simulink model "Assignment1"  (R2020a)
settings: Solver=FixedStepAuto  StartTime=0.0  StopTime=5  FixedStep=1e-3  RelTol=1e-3  EnableMultiTasking=on
model workspace (MAT data in the model file):
  ATR_CMP_REF_PWM_PERCENTAGE = 50
  PACING_REF_PWM_DUTY_PERCENTAGE = 50
  VENT_CMP_REF_PWM_PERCENTAGE = 50
undefined symbols (not defined in the file): A0, A1, D0, D1, D10, D11, D12, D13, D2, D3, D4, D5, D6, D7, D8, D9, magnitude, PTA0, PTA1, PTA2, PTB2, PTB23, PTB3, PTB9, PTC16, PTC17, PTC2, PTC3, PTC4, PTD0, PTD1, PTD2, PTD3
libraries: frdmk64flib x22, etargetslib x18, dspstat3 x1
settings Model: ExtModeTrigDuration=5  OrderedModelArguments=off  Creator=John  LastModifiedBy=changhaibian
settings OptimizationCC: EnhancedBackFolding=on  PassReuseOutputArgsAs=Individual arguments  ZeroExternalMemoryAtStartup=off  ZeroInternalMemoryAtStartup=off  MaxStackSize=64  OptimizeBlockOrder=speed  DifferentSizesBufferReuse=on  OptimizationCustomize=off  EfficientTunableParamExpr=on
settings DebuggingCC: ParameterTunabilityLossMsg=error
settings HardwareCC: ProdBitPerPointer=32  ProdBitPerSizeT=32  ProdBitPerPtrDiffT=32  ProdLargestAtomicInteger=Long  ProdLargestAtomicFloat=Double  ProdWordSize=32  ProdHWDeviceType=ARM Compatible->ARM Cortex
settings SFSimCC: MATLABDynamicMemAlloc=off
settings RTWCC: SystemTargetFile=ert.tlc  HardwareBoard=NXP FRDM-K64F  TemplateMakefile=ert_default_tmf  Toolchain=GNU Tools for ARM Embedded Processors
settings CodeAppCC: ForceParamTrailComments=on  IgnoreCustomStorageClasses=off  OperatorAnnotations=on  SimulinkDataObjDesc=on  SFDataObjDesc=on  InsertBlockDesc=on

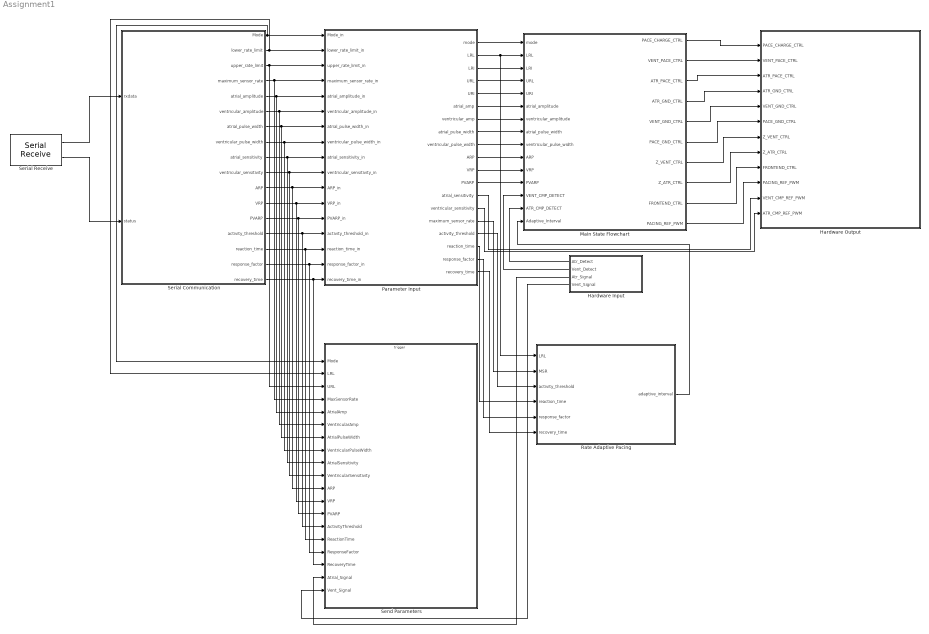
== system Assignment1 ==
  Hardware Input : Subsystem
      settings: PortSchema="{\"entries\":[{\"content\":{\"sides\":[{\"content\":{\"connectorIds\":[\"Out1\",\"Out2\",\"Out3\",\"Out4\"]},\"type\":\"ConnectorPlacement.EquallySpacedRectSide\",\"uuid\":\"5cee9ea6-bf5d-4625-bfce-39977475e911\"},{\"content\":{\"connectorIds\":[],\"side\":\"RIGHT\"},\"type\":\"ConnectorPlacement.EquallySpacedRectSide\",\"uuid\":\"d8f9e342-4161-4713-ba8e-977d0ac6df9e\"},{\"content\":{\"connectorIds\":[],\"side\":\"TOP\"},\"type\":\"ConnectorPlacement.EquallySpacedRectSide\",\"uuid\":\"5d530249-14f9-42e8-9a17-4b94b2159c30\"}]},\"type\":\"ConnectorPlacement.EquallySpacedConnector\",\"uuid\":\"d67ebefe-f0b3-4c88-9ae8-796034241cb9\"}],\"packageUris\":[\"http://schema.mathworks.com/mf0/Connector/19700101\"],\"version\":\"1.0\"}"
  Hardware Output : Subsystem
  Main State Flowchart : Stateflow chart  TreatAsAtomicUnit=on
  Parameter Input : Subsystem
  Rate Adaptive Pacing : Subsystem
  Send Parameters : Subsystem  TreatAsAtomicUnit=on
  Serial Communication : Stateflow chart  TreatAsAtomicUnit=on
  Serial Receive : frdmk64flib/Serial Receive  SCIModule=0  Baudrate=uint32(9600)  Parity=None  StopBits=1  HardwareFlowControl=None  ByteOrder=LittleEndian  DataType=uint8  DataLength=11  BlockingMode=off  OutputStatus=on  SampleTime=-1
  wires:
  Parameter Input/1(mode) -> Main State Flowchart/1(mode)
  Main State Flowchart/10(PACING_REF_PWM) -> Hardware Output/10(PACING_REF_PWM)
  Parameter Input/8(atrial_pulse_width) -> Main State Flowchart/8(atrial_pulse_width)
  Parameter Input/9(ventricular_pulse_width) -> Main State Flowchart/9(ventricular_pulse_width)
  Main State Flowchart/7(Z_VENT_CTRL) -> Hardware Output/7(Z_VENT_CTRL)
  Main State Flowchart/4(ATR_GND_CTRL) -> Hardware Output/4(ATR_GND_CTRL)
  Main State Flowchart/3(ATR_PACE_CTRL) -> Hardware Output/3(ATR_PACE_CTRL)
  Main State Flowchart/5(VENT_GND_CTRL) -> Hardware Output/5(VENT_GND_CTRL)
  Main State Flowchart/2(VENT_PACE_CTRL) -> Hardware Output/2(VENT_PACE_CTRL)
  Main State Flowchart/1(PACE_CHARGE_CTRL) -> Hardware Output/1(PACE_CHARGE_CTRL)
  Main State Flowchart/9(FRONTEND_CTRL) -> Hardware Output/9(FRONTEND_CTRL)
  Parameter Input/2(LRL) -> Rate Adaptive Pacing/1(LRL), Main State Flowchart/2(LRL)
  Parameter Input/10(ARP) -> Main State Flowchart/10(ARP)
  Parameter Input/11(VRP) -> Main State Flowchart/11(VRP)
  Parameter Input/6(atrial_amp) -> Main State Flowchart/6(atrial_amplitude)
  Parameter Input/3(LRI) -> Main State Flowchart/3(LRI)
  Parameter Input/4(URL) -> Main State Flowchart/4(URL)
  Parameter Input/5(URI) -> Main State Flowchart/5(URI)
  Serial Receive/1 -> Serial Communication/1(rxdata)
  Serial Receive/2 -> Serial Communication/2(status)
  Serial Communication/1(Mode) -> Send Parameters/1(Mode), Parameter Input/1(Mode_in)
  Serial Communication/2(lower_rate_limit) -> Send Parameters/2(LRL), Parameter Input/2(lower_rate_limit_in)
  Serial Communication/3(upper_rate_limit) -> Parameter Input/3(upper_rate_limit_in), Send Parameters/3(URL)
  Serial Communication/4(maximum_sensor_rate) -> Send Parameters/4(MaxSensorRate), Parameter Input/4(maximum_sensor_rate_in)
  Serial Communication/5(atrial_amplitude) -> Send Parameters/5(AtrialAmp), Parameter Input/5(atrial_amplitude_in)
  Serial Communication/6(ventricular_amplitude) -> Send Parameters/6(VentricularAmp), Parameter Input/6(ventricular_amplitude_in)
  Serial Communication/7(atrial_pulse_width) -> Send Parameters/7(AtrialPulseWidth), Parameter Input/7(atrial_pulse_width_in)
  Serial Communication/8(ventricular_pulse_width) -> Send Parameters/8(VentricularPulseWidth), Parameter Input/8(ventricular_pulse_width_in)
  Serial Communication/9(atrial_sensitivity) -> Send Parameters/9(AtrialSensitivity), Parameter Input/9(atrial_sensitivity_in)
  Serial Communication/10(ventricular_sensitivity) -> Send Parameters/10(VentricularSensitivity), Parameter Input/10(ventricular_sensitivity_in)
  Serial Communication/11(ARP) -> Send Parameters/11(ARP), Parameter Input/11(ARP_in)
  Serial Communication/12(VRP) -> Send Parameters/12(VRP), Parameter Input/12(VRP_in)
  Serial Communication/13(PVARP) -> Send Parameters/13(PVARP), Parameter Input/13(PVARP_in)
  Serial Communication/14(activity_threshold) -> Send Parameters/14(ActivityThreshold), Parameter Input/14(activity_threshold_in)
  Serial Communication/15(reaction_time) -> Send Parameters/15(ReactionTime), Parameter Input/15(reaction_time_in)
  Serial Communication/16(response_factor) -> Send Parameters/16(ResponseFactor), Parameter Input/16(response_factor_in)
  Serial Communication/17(recovery_time) -> Send Parameters/17(RecoveryTime), Parameter Input/17(recovery_time_in)
  Parameter Input/7(ventricular_amp) -> Main State Flowchart/7(ventricular_amplitude)
  Parameter Input/12(PVARP) -> Main State Flowchart/12(PVARP)
  Hardware Input/1(Atr_Detect) -> Main State Flowchart/14(ATR_CMP_DETECT)
  Hardware Input/2(Vent_Detect) -> Main State Flowchart/13(VENT_CMP_DETECT)
  Rate Adaptive Pacing/1(adaptive_interval) -> Main State Flowchart/15(Adaptive_Interval)
  Parameter Input/13(atrial_sensitivity) -> Hardware Output/11(VENT_CMP_REF_PWM)
  Parameter Input/14(ventricular_sensitivity) -> Hardware Output/12(ATR_CMP_REF_PWM)
  Hardware Input/3(Atr_Signal) -> Send Parameters/18(Atrial_Signal)
  Hardware Input/4(Vent_Signal) -> Send Parameters/19(Vent_Signal)
  Parameter Input/19(recovery_time) -> Rate Adaptive Pacing/6(recovery_time)
  Parameter Input/18(response_factor) -> Rate Adaptive Pacing/5(response_factor)
  Parameter Input/17(reaction_time) -> Rate Adaptive Pacing/4(reaction_time)
  Parameter Input/16(activity_threshold) -> Rate Adaptive Pacing/3(activity_threshold)
  Parameter Input/15(maximum_sensor_rate) -> Rate Adaptive Pacing/2(MSR)
  Main State Flowchart/6(PACE_GND_CTRL) -> Hardware Output/6(PACE_GND_CTRL)
  Main State Flowchart/8(Z_ATR_CTRL) -> Hardware Output/8(Z_ATR_CTRL)

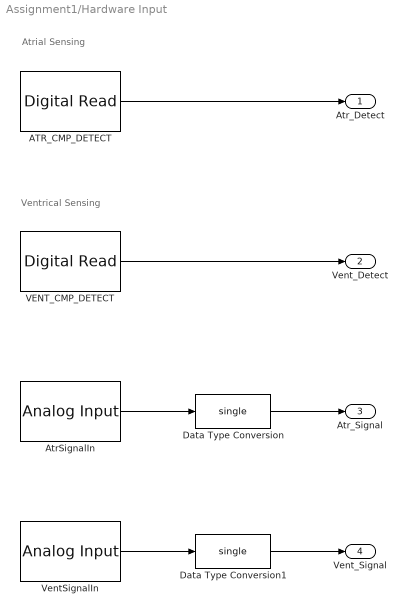
== system Assignment1/Hardware Input ==
  note: Ventrical Sensing
  note: Atrial Sensing
  ATR_CMP_DETECT : frdmk64flib/Digital Read  Whichpin=PTC16 (D0)  SampleTime=-1
  AtrSignalIn : frdmk64flib/Analog Input  Whichpin=PTB2 (A0)  SampleTime=-1
  Data Type Conversion : DataTypeConversion  OutDataTypeStr=single
  Data Type Conversion1 : DataTypeConversion  OutDataTypeStr=single
  VENT_CMP_DETECT : frdmk64flib/Digital Read  Whichpin=PTC17 (D1)  SampleTime=-1
  VentSignalIn : frdmk64flib/Analog Input  Whichpin=PTB3 (A1)  SampleTime=-1
  Atr_Detect : Outport
  Vent_Detect : Outport  Port=2
  Atr_Signal : Outport  Port=3  OutDataTypeStr=single
  Vent_Signal : Outport  Port=4  OutDataTypeStr=single
  wires:
  ATR_CMP_DETECT/1 -> Atr_Detect/1
  VENT_CMP_DETECT/1 -> Vent_Detect/1
  AtrSignalIn/1 -> Data Type Conversion/1
  Data Type Conversion/1 -> Atr_Signal/1
  VentSignalIn/1 -> Data Type Conversion1/1
  Data Type Conversion1/1 -> Vent_Signal/1

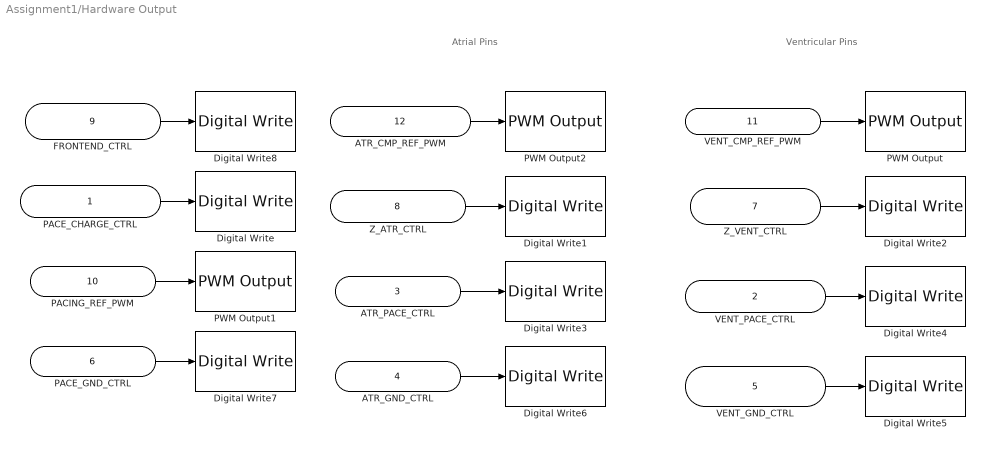
== system Assignment1/Hardware Output ==
  note: Ventricular Pins
  note: Atrial Pins
  PACE_CHARGE_CTRL : Inport
  VENT_PACE_CTRL : Inport  Port=2
  ATR_PACE_CTRL : Inport  Port=3
  ATR_GND_CTRL : Inport  Port=4
  VENT_GND_CTRL : Inport  Port=5
  PACE_GND_CTRL : Inport  Port=6
  Z_VENT_CTRL : Inport  Port=7
  Z_ATR_CTRL : Inport  Port=8
  FRONTEND_CTRL : Inport  Port=9
  PACING_REF_PWM : Inport  Port=10
  VENT_CMP_REF_PWM : Inport  Port=11
  ATR_CMP_REF_PWM : Inport  Port=12
  Digital Write : frdmk64flib/Digital Write  Whichpin=PTB9 (D2)
  Digital Write1 : frdmk64flib/Digital Write  Whichpin=PTB23 (D4)
  Digital Write2 : frdmk64flib/Digital Write  Whichpin=PTC3 (D7)
  Digital Write3 : frdmk64flib/Digital Write  Whichpin=PTA0 (D8)
  Digital Write4 : frdmk64flib/Digital Write  Whichpin=PTC4 (D9)
  Digital Write5 : frdmk64flib/Digital Write  Whichpin=PTD3 (D12)
  Digital Write6 : frdmk64flib/Digital Write  Whichpin=PTD2 (D11)
  Digital Write7 : frdmk64flib/Digital Write  Whichpin=PTD0 (D10)
  Digital Write8 : frdmk64flib/Digital Write  Whichpin=PTD1 (D13)
  PWM Output : frdmk64flib/PWM Output  Whichpin=PTC2 (D6)  InitialFrequency=2000  InitialDutyCycle=0
  PWM Output1 : frdmk64flib/PWM Output  Whichpin=PTA2 (D5)  InitialFrequency=2000  InitialDutyCycle=0
  PWM Output2 : frdmk64flib/PWM Output  Whichpin=PTA1 (D3)  InitialFrequency=2000  InitialDutyCycle=0
  wires:
  VENT_PACE_CTRL/1 -> Digital Write4/1
  Z_ATR_CTRL/1 -> Digital Write1/1
  PACE_GND_CTRL/1 -> Digital Write7/1
  FRONTEND_CTRL/1 -> Digital Write8/1
  PACING_REF_PWM/1 -> PWM Output1/1
  VENT_CMP_REF_PWM/1 -> PWM Output/1
  PACE_CHARGE_CTRL/1 -> Digital Write/1
  Z_VENT_CTRL/1 -> Digital Write2/1
  VENT_GND_CTRL/1 -> Digital Write5/1
  ATR_PACE_CTRL/1 -> Digital Write3/1
  ATR_CMP_REF_PWM/1 -> PWM Output2/1
  ATR_GND_CTRL/1 -> Digital Write6/1

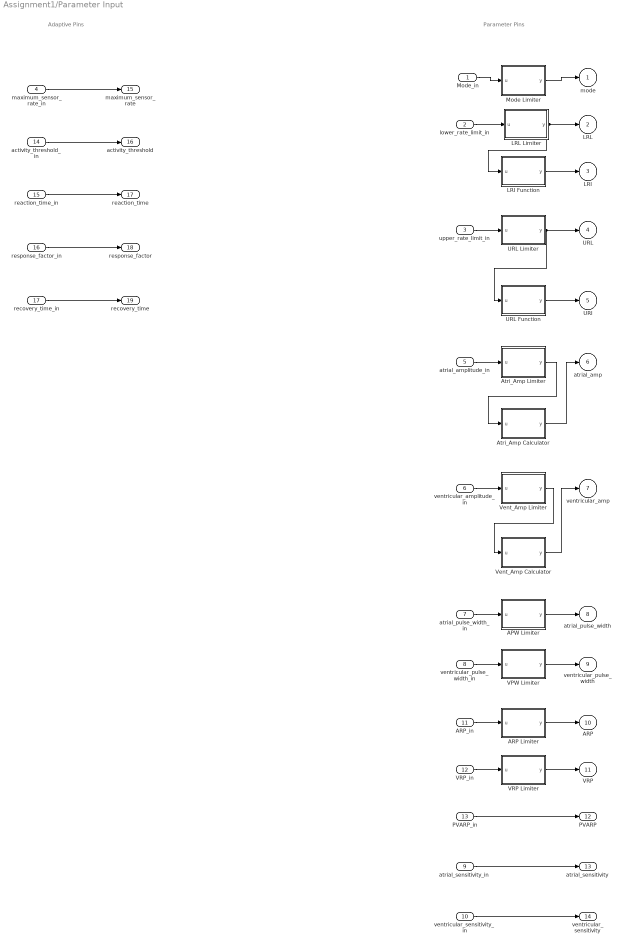
== system Assignment1/Parameter Input ==
  note: Adaptive Pins
  note: Parameter Pins
  Mode_in : Inport  OutDataTypeStr=uint8
  lower_rate_limit_in : Inport  Port=2  OutDataTypeStr=single
  upper_rate_limit_in : Inport  Port=3  OutDataTypeStr=single
  maximum_sensor_rate_in : Inport  Port=4  OutDataTypeStr=single
  atrial_amplitude_in : Inport  Port=5  OutDataTypeStr=single  Unit=V
  ventricular_amplitude_in : Inport  Port=6  OutDataTypeStr=single  Unit=V
  atrial_pulse_width_in : Inport  Port=7  OutDataTypeStr=single  Unit=ms  LockScale=on
  ventricular_pulse_width_in : Inport  Port=8  OutDataTypeStr=single  Unit=ms
  atrial_sensitivity_in : Inport  Port=9  OutDataTypeStr=single  Unit=mV
  ventricular_sensitivity_in : Inport  Port=10  OutDataTypeStr=single  Unit=mV
  ARP_in : Inport  Port=11  OutDataTypeStr=single  Unit=ms
  VRP_in : Inport  Port=12  OutDataTypeStr=single  Unit=ms
  PVARP_in : Inport  Port=13  OutDataTypeStr=uint16  Unit=ms
  activity_threshold_in : Inport  Port=14  OutDataTypeStr=single
  reaction_time_in : Inport  Port=15  OutDataTypeStr=single  Unit=s
  response_factor_in : Inport  Port=16  OutDataTypeStr=single
  recovery_time_in : Inport  Port=17  OutDataTypeStr=single  Unit=s
  APW Limiter : MATLAB Function  TreatAsAtomicUnit=on
  ARP Limiter : MATLAB Function  TreatAsAtomicUnit=on
  Atri_Amp Calculator : MATLAB Function  TreatAsAtomicUnit=on
  Atri_Amp Limiter : MATLAB Function  TreatAsAtomicUnit=on
  LRI Function : MATLAB Function  TreatAsAtomicUnit=on
  LRL Limiter : MATLAB Function  TreatAsAtomicUnit=on
  Mode Limiter : MATLAB Function  TreatAsAtomicUnit=on
  URL Function : MATLAB Function  TreatAsAtomicUnit=on
  URL Limiter : MATLAB Function  TreatAsAtomicUnit=on
  VPW Limiter : MATLAB Function  TreatAsAtomicUnit=on
  VRP Limiter : MATLAB Function  TreatAsAtomicUnit=on
  Vent_Amp Calculator : MATLAB Function  TreatAsAtomicUnit=on
  Vent_Amp Limiter : MATLAB Function  TreatAsAtomicUnit=on
  mode : Outport  OutDataTypeStr=uint8
  LRL : Outport  Port=2  OutDataTypeStr=single
  LRI : Outport  Port=3  OutDataTypeStr=single
  URL : Outport  Port=4  OutDataTypeStr=single
  URI : Outport  Port=5  OutDataTypeStr=single
  atrial_amp : Outport  Port=6  OutDataTypeStr=single
  ventricular_amp : Outport  Port=7  OutDataTypeStr=single
  atrial_pulse_width : Outport  Port=8  OutDataTypeStr=single
  ventricular_pulse_width : Outport  Port=9  OutDataTypeStr=single
  ARP : Outport  Port=10  OutDataTypeStr=single
  VRP : Outport  Port=11  OutDataTypeStr=single
  PVARP : Outport  Port=12  OutDataTypeStr=uint16
  atrial_sensitivity : Outport  Port=13  OutDataTypeStr=single
  ventricular_sensitivity : Outport  Port=14  OutDataTypeStr=single
  maximum_sensor_rate : Outport  Port=15  OutDataTypeStr=single
  activity_threshold : Outport  Port=16  OutDataTypeStr=single
  reaction_time : Outport  Port=17  OutDataTypeStr=single
  response_factor : Outport  Port=18  OutDataTypeStr=single
  recovery_time : Outport  Port=19  OutDataTypeStr=single
  wires:
  Mode Limiter/1(y) -> mode/1
  APW Limiter/1(y) -> atrial_pulse_width/1
  VPW Limiter/1(y) -> ventricular_pulse_width/1
  LRI Function/1(y) -> LRI/1
  VRP Limiter/1(y) -> VRP/1
  VRP_in/1 -> VRP Limiter/1(u)
  ARP Limiter/1(y) -> ARP/1
  LRL Limiter/1(y) -> LRI Function/1(u), LRL/1
  Atri_Amp Limiter/1(y) -> Atri_Amp Calculator/1(u)
  URL Function/1(y) -> URI/1
  Mode_in/1 -> Mode Limiter/1(u)
  lower_rate_limit_in/1 -> LRL Limiter/1(u)
  upper_rate_limit_in/1 -> URL Limiter/1(u)
  atrial_amplitude_in/1 -> Atri_Amp Limiter/1(u)
  Vent_Amp Limiter/1(y) -> Vent_Amp Calculator/1(u)
  ventricular_amplitude_in/1 -> Vent_Amp Limiter/1(u)
  maximum_sensor_rate_in/1 -> maximum_sensor_rate/1
  activity_threshold_in/1 -> activity_threshold/1
  reaction_time_in/1 -> reaction_time/1
  response_factor_in/1 -> response_factor/1
  recovery_time_in/1 -> recovery_time/1
  atrial_pulse_width_in/1 -> APW Limiter/1(u)
  ventricular_pulse_width_in/1 -> VPW Limiter/1(u)
  Atri_Amp Calculator/1(y) -> atrial_amp/1
  Vent_Amp Calculator/1(y) -> ventricular_amp/1
  URL Limiter/1(y) -> URL Function/1(u), URL/1
  ARP_in/1 -> ARP Limiter/1(u)
  PVARP_in/1 -> PVARP/1
  atrial_sensitivity_in/1 -> atrial_sensitivity/1
  ventricular_sensitivity_in/1 -> ventricular_sensitivity/1

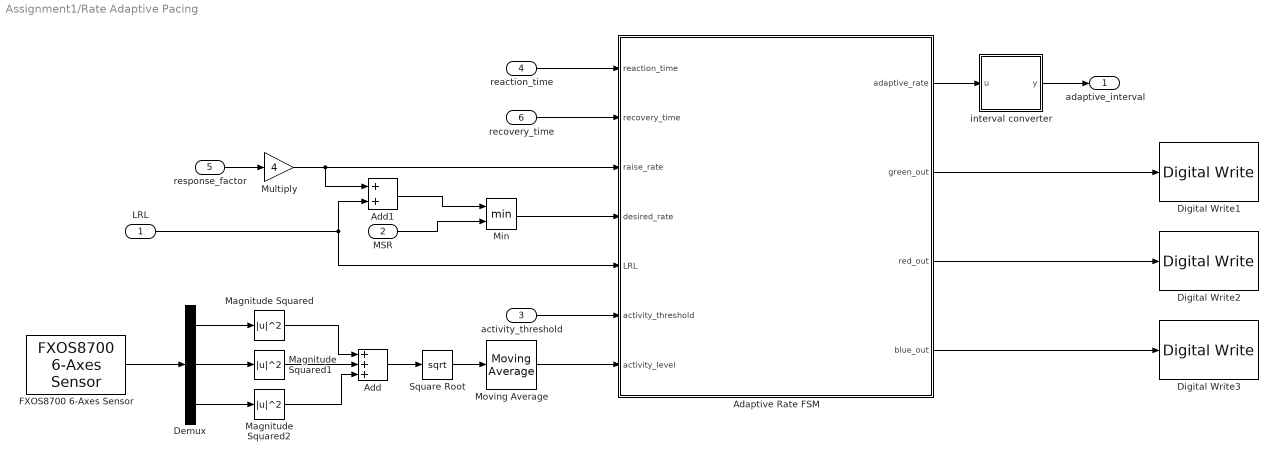
== system Assignment1/Rate Adaptive Pacing ==
  LRL : Inport  OutDataTypeStr=single
  MSR : Inport  Port=2  OutDataTypeStr=single
  activity_threshold : Inport  Port=3  OutDataTypeStr=single
  reaction_time : Inport  Port=4  OutDataTypeStr=single
  response_factor : Inport  Port=5  OutDataTypeStr=single
  recovery_time : Inport  Port=6  OutDataTypeStr=single
  Adaptive Rate FSM : Stateflow chart  TreatAsAtomicUnit=on
      settings: PortSchema="{\"entries\":[{\"content\":{\"sides\":[{\"content\":{\"connectorIds\":[\"In1\",\"In2\",\"In5\",\"In7\",\"In4\",\"In3\",\"In6\"]},\"type\":\"ConnectorPlacement.EquallySpacedRectSide\",\"uuid\":\"ac5b5a9a-baa0-451d-a6e3-39214b5ee711\"},{\"content\":{\"connectorIds\":[\"Out1\",\"Out2\",\"Out3\",\"Out4\"],\"side\":\"RIGHT\"},\"type\":\"ConnectorPlacement.EquallySpacedRectSide\",\"uuid\":\"f0426f16-b598-4be9-afee-34b2a98f2478\"},{\"content\":{\"connectorIds\":[],\"side\":\"TOP\"},\"type\":\"ConnectorPlacement.EquallySpacedRectSide\",\"uuid\":\"5575c0ab-c844-4404-9f77-8963aaae3938\"}]},\"type\":\"ConnectorPlacement.EquallySpacedConnector\",\"uuid\":\"4a585840-eacd-4a9f-bbb3-6604f7385cf9\"}],\"packageUris\":[\"http://schema.mathworks.com/mf0/Connector/19700101\"],\"version\":\"1.0\"}"
  Add : Sum  Inputs=+++
  Add1 : Sum  OutDataTypeStr=single  RndMeth=Nearest
  Demux : Demux  Outputs=3
  Digital Write1 : frdmk64flib/Digital Write  Whichpin=GREEN_LED
  Digital Write2 : frdmk64flib/Digital Write  Whichpin=RED_LED
  Digital Write3 : frdmk64flib/Digital Write  Whichpin=BLUE_LED
  FXOS8700 6-Axes Sensor : frdmk64flib/FXOS8700 6-Axes Sensor  Activesensor=Accelerometer only  ODR=800Hz  HybridODR=400Hz  Accelfullrange=-4g to +4g  SampleTime=-1
  Magnitude Squared : Math  Operator=magnitude^2  SaturateOnIntegerOverflow=on
  Magnitude Squared1 : Math  Operator=magnitude^2  SaturateOnIntegerOverflow=on
  Magnitude Squared2 : Math  Operator=magnitude^2  SaturateOnIntegerOverflow=on
  Min : MinMax  Inputs=2  OutDataTypeStr=single
  Moving Average : dspstat3/Moving Average  Method=Sliding window  ForgettingFactorPort=off  SpecifyWindowLength=on  WindowLength=4  ForgettingFactor=0.9  SimulateUsing=Code generation
  Multiply : Gain  Gain=4  ParamDataTypeStr=uint8  OutDataTypeStr=single
  Square Root : Sqrt  SaturateOnIntegerOverflow=on
  interval converter : MATLAB Function  TreatAsAtomicUnit=on
  adaptive_interval : Outport  OutDataTypeStr=single
  wires:
  Adaptive Rate FSM/1(adaptive_rate) -> interval converter/1(u)
  LRL/1 -> Adaptive Rate FSM/4(LRL), Add1/2
  FXOS8700 6-Axes Sensor/1 -> Demux/1
  Demux/1 -> Magnitude Squared/1
  Moving Average/1 -> Adaptive Rate FSM/6(activity_level)
  Square Root/1 -> Moving Average/1
  Add/1 -> Square Root/1
  Demux/3 -> Magnitude Squared2/1
  Demux/2 -> Magnitude Squared1/1
  Magnitude Squared1/1 -> Add/2
  Magnitude Squared/1 -> Add/1
  Magnitude Squared2/1 -> Add/3
  activity_threshold/1 -> Adaptive Rate FSM/3(activity_threshold)
  interval converter/1(y) -> adaptive_interval/1
  reaction_time/1 -> Adaptive Rate FSM/1(reaction_time)
  recovery_time/1 -> Adaptive Rate FSM/2(recovery_time)
  MSR/1 -> Min/2
  Adaptive Rate FSM/2(green_out) -> Digital Write1/1
  Adaptive Rate FSM/3(red_out) -> Digital Write2/1
  Adaptive Rate FSM/4(blue_out) -> Digital Write3/1
  Add1/1 -> Min/1
  Min/1 -> Adaptive Rate FSM/7(desired_rate)
  response_factor/1 -> Multiply/1
  Multiply/1 -> Add1/1, Adaptive Rate FSM/5(raise_rate)

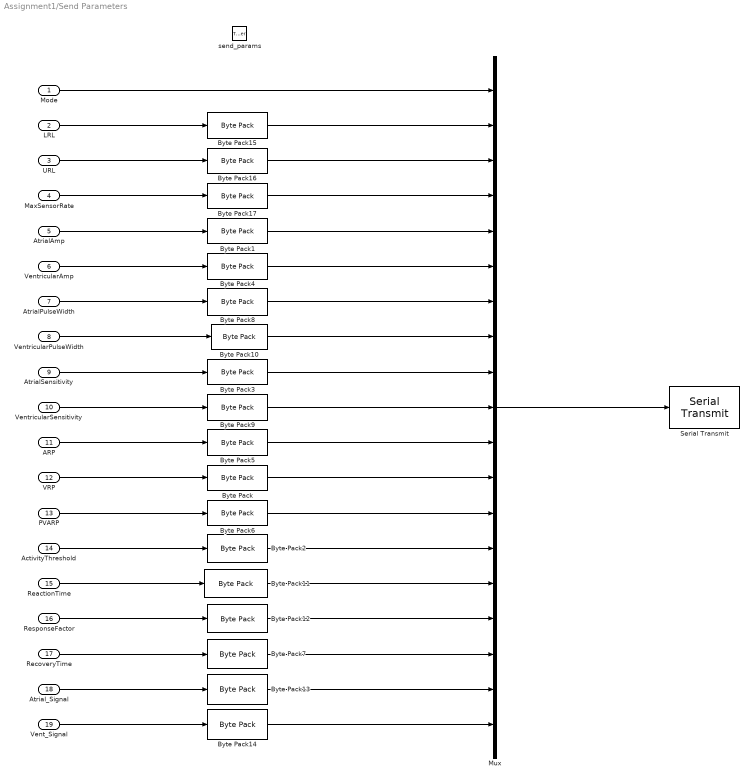
== system Assignment1/Send Parameters ==
  Mode : Inport  OutDataTypeStr=uint8
  LRL : Inport  Port=2  OutDataTypeStr=single
  URL : Inport  Port=3  OutDataTypeStr=single
  MaxSensorRate : Inport  Port=4  OutDataTypeStr=single
  AtrialAmp : Inport  Port=5  OutDataTypeStr=single
  VentricularAmp : Inport  Port=6  OutDataTypeStr=single
  AtrialPulseWidth : Inport  Port=7  OutDataTypeStr=single
  VentricularPulseWidth : Inport  Port=8  OutDataTypeStr=single
  AtrialSensitivity : Inport  Port=9  OutDataTypeStr=single
  VentricularSensitivity : Inport  Port=10  OutDataTypeStr=single
  ARP : Inport  Port=11  OutDataTypeStr=single
  VRP : Inport  Port=12  OutDataTypeStr=single
  PVARP : Inport  Port=13  OutDataTypeStr=uint16
  ActivityThreshold : Inport  Port=14  OutDataTypeStr=single
  ReactionTime : Inport  Port=15  OutDataTypeStr=single
  ResponseFactor : Inport  Port=16  OutDataTypeStr=single
  RecoveryTime : Inport  Port=17  OutDataTypeStr=single
  Atrial_Signal : Inport  Port=18  OutDataTypeStr=single
  Vent_Signal : Inport  Port=19  OutDataTypeStr=single
  send_params : TriggerPort  TriggerType=function-call  IsSimulinkFunction=on  FunctionName=send_params  VariantControl=Variant
  Byte Pack{,1..5,7..17} (17 alike) : etargetslib/Byte Pack  datatypes={'single'}  byteAlign=1
  Byte Pack6 : etargetslib/Byte Pack  datatypes={'uint16'}  byteAlign=1
  Mux : Mux  Inputs=19
  Serial Transmit : frdmk64flib/Serial Transmit  SCIModule=0  Baudrate=uint32(9600)  Parity=None  StopBits=1  HardwareFlowControl=None  ByteOrder=LittleEndian  BlockingMode=on  OutputStatus=off
  wires:
  Byte Pack9/1 -> Mux/10
  Mode/1 -> Mux/1
  ARP/1 -> Byte Pack5/1
  VentricularAmp/1 -> Byte Pack4/1
  VentricularSensitivity/1 -> Byte Pack9/1
  AtrialSensitivity/1 -> Byte Pack3/1
  VRP/1 -> Byte Pack/1
  AtrialAmp/1 -> Byte Pack1/1
  Byte Pack6/1 -> Mux/13
  PVARP/1 -> Byte Pack6/1
  Byte Pack1/1 -> Mux/5
  Byte Pack4/1 -> Mux/6
  Byte Pack3/1 -> Mux/9
  Byte Pack5/1 -> Mux/11
  Byte Pack/1 -> Mux/12
  ActivityThreshold/1 -> Byte Pack2/1
  Byte Pack2/1 -> Mux/14
  RecoveryTime/1 -> Byte Pack7/1
  Byte Pack7/1 -> Mux/17
  Mux/1 -> Serial Transmit/1
  AtrialPulseWidth/1 -> Byte Pack8/1
  Byte Pack8/1 -> Mux/7
  VentricularPulseWidth/1 -> Byte Pack10/1
  Byte Pack10/1 -> Mux/8
  ReactionTime/1 -> Byte Pack11/1
  Byte Pack11/1 -> Mux/15
  ResponseFactor/1 -> Byte Pack12/1
  Byte Pack12/1 -> Mux/16
  Atrial_Signal/1 -> Byte Pack13/1
  Byte Pack13/1 -> Mux/18
  Vent_Signal/1 -> Byte Pack14/1
  Byte Pack14/1 -> Mux/19
  LRL/1 -> Byte Pack15/1
  Byte Pack15/1 -> Mux/2
  URL/1 -> Byte Pack16/1
  Byte Pack16/1 -> Mux/3
  MaxSensorRate/1 -> Byte Pack17/1
  Byte Pack17/1 -> Mux/4

== matlab function Assignment1/Parameter Input/APW Limiter ==
  data: u input; y output
function y = fcn(u)
    if u >= 20
       u = single(20);
    elseif u <= 0
        u = single(0);
    end
y = u;

== matlab function Assignment1/Parameter Input/Mode Limiter ==
  data: u input; y output
function y = fcn(u)
    if u > 6
       u = uint8(0);
    elseif u < 1
       u = uint8(0);
    end
y = u;

== stateflow chart Assignment1/Main State Flowchart ==
  state AOOR
    state AOOR_Charge
      entry:
      PACING_REF_PWM = atrial_amplitude;
      ATR_CMP_REF_PWM = 70;
      PACE_CHARGE_CTRL = 1;
      PACE_GND_CTRL = 1;
      ATR_PACE_CTRL = 0;
      ATR_GND_CTRL = 1;
      VENT_PACE_CTRL = 0;
      VENT_GND_CTRL = 0;
      Z_ATR_CTRL = 0;
      Z_VENT_CTRL =0;
      FRONTEND_CTRL = 0;
    state Atrial_Pacing
      entry:
      PACING_REF_PWM = atrial_amplitude;
      ATR_CMP_REF_PWM = 70;
      PACE_CHARGE_CTRL = 0;
      PACE_GND_CTRL = 1;
      ATR_PACE_CTRL = 1;
      ATR_GND_CTRL = 0;
      VENT_PACE_CTRL = 0;
      VENT_GND_CTRL = 0;
      Z_ATR_CTRL = 0;
      Z_VENT_CTRL = 0;
    (default) -> AOOR_Charge
    AOOR_Charge -> AOOR.Atrial_Pacing : [after(Adaptive_Interval - atrial_pulse_width,msec)]
    AOOR.Atrial_Pacing -> AOOR_Charge : [after(atrial_pulse_width,msec)]
  state AAI
    state delay
    state AOO_Charge
      entry:
      PACING_REF_PWM = atrial_amplitude;
      ATR_CMP_REF_PWM = 70;
      PACE_CHARGE_CTRL = 1;
      PACE_GND_CTRL = 1;
      ATR_PACE_CTRL = 0;
      ATR_GND_CTRL = 1;
      VENT_PACE_CTRL = 0;
      VENT_GND_CTRL = 0;
      Z_ATR_CTRL = 0;
      Z_VENT_CTRL =0;
      FRONTEND_CTRL = 0;
    state sense
      entry:
      FRONTEND_CTRL = 1;
    state inhibited_ARP
    state Atrial_Pacing
      entry:
      PACING_REF_PWM = atrial_amplitude;
      ATR_CMP_REF_PWM = 70;
      PACE_CHARGE_CTRL = 0;
      PACE_GND_CTRL = 1;
      ATR_PACE_CTRL = 1;
      ATR_GND_CTRL = 0;
      VENT_PACE_CTRL = 0;
      VENT_GND_CTRL = 0;
      Z_ATR_CTRL = 0;
      Z_VENT_CTRL = 0;
    (default) -> AAI.AOO_Charge
    AAI.delay -> AAI.sense : [after(ARP,msec)]
    AAI.sense -> AAI.delay [order 1] : [ATR_CMP_DETECT == 1]
    AAI.AOO_Charge -> AAI.inhibited_ARP
    AAI.inhibited_ARP -> AAI.sense : [after(ARP,msec)]
    AAI.sense -> AAI.Atrial_Pacing [order 2] : [after(LRI - ARP,msec) && ATR_CMP_DETECT == 0]
    AAI.Atrial_Pacing -> AAI.AOO_Charge : [after(atrial_pulse_width,msec)]
  state AAIR
    state delay
    state AOO_Charge
      entry:
      PACING_REF_PWM = atrial_amplitude;
      ATR_CMP_REF_PWM = 70;
      PACE_CHARGE_CTRL = 1;
      PACE_GND_CTRL = 1;
      ATR_PACE_CTRL = 0;
      ATR_GND_CTRL = 1;
      VENT_PACE_CTRL = 0;
      VENT_GND_CTRL = 0;
      Z_ATR_CTRL = 0;
      Z_VENT_CTRL =0;
      FRONTEND_CTRL = 0;
    state sense
      entry:
      FRONTEND_CTRL = 1;
    state inhibited_ARP
    state Atrial_Pacing
      entry:
      PACING_REF_PWM = atrial_amplitude;
      ATR_CMP_REF_PWM = 70;
      PACE_CHARGE_CTRL = 0;
      PACE_GND_CTRL = 1;
      ATR_PACE_CTRL = 1;
      ATR_GND_CTRL = 0;
      VENT_PACE_CTRL = 0;
      VENT_GND_CTRL = 0;
      Z_ATR_CTRL = 0;
      Z_VENT_CTRL = 0;
    (default) -> AAIR.AOO_Charge
    AAIR.delay -> AAIR.sense : [after(ARP,msec)]
    AAIR.sense -> AAIR.delay [order 1] : [ATR_CMP_DETECT == 1]
    AAIR.AOO_Charge -> AAIR.inhibited_ARP
    AAIR.inhibited_ARP -> AAIR.sense : [after(ARP,msec)]
    AAIR.sense -> AAIR.Atrial_Pacing [order 2] : [after(Adaptive_Interval - ARP,msec) && ATR_CMP_DETECT == 0]
    AAIR.Atrial_Pacing -> AAIR.AOO_Charge : [after(atrial_pulse_width,msec)]
  state VVI
    state delay
    state VVI_Charge
      entry:
      PACING_REF_PWM = atrial_amplitude;
      VENT_CMP_REF_PWM = 70;
      PACE_CHARGE_CTRL = 1;
      PACE_GND_CTRL = 1;
      ATR_PACE_CTRL = 0;
      ATR_GND_CTRL = 0;
      VENT_PACE_CTRL = 0;
      VENT_GND_CTRL = 1;
      Z_ATR_CTRL = 0;
      Z_VENT_CTRL =0;
    state sense
      entry:
      FRONTEND_CTRL = 1;
    state inhibited_VRP
    state Ventricular_Pacing
      entry:
      PACING_REF_PWM = atrial_amplitude;
      VENT_CMP_REF_PWM = 70;
      PACE_CHARGE_CTRL = 0;
      PACE_GND_CTRL = 1;
      ATR_PACE_CTRL = 0;
      ATR_GND_CTRL = 0;
      Z_ATR_CTRL = 0;
      Z_VENT_CTRL = 0;
      VENT_PACE_CTRL = 1;
      VENT_GND_CTRL = 0;
    VVI.delay -> VVI.sense : [after(VRP - ventricular_pulse_width,msec)]
    (default) -> VVI.VVI_Charge
    VVI.sense -> VVI.delay [order 1] : [VENT_CMP_DETECT == 1]
    VVI.VVI_Charge -> VVI.inhibited_VRP
    VVI.inhibited_VRP -> VVI.sense : [after(VRP - ventricular_pulse_width,msec)]
    VVI.sense -> VVI.Ventricular_Pacing [order 2] : [after(LRI - VRP,msec) && VENT_CMP_DETECT == 0]
    VVI.Ventricular_Pacing -> VVI.VVI_Charge : [after(ventricular_pulse_width,msec)]
  state AOO
    state AOO_Charge
      entry:
      PACING_REF_PWM = atrial_amplitude;
      ATR_CMP_REF_PWM = 70;
      PACE_CHARGE_CTRL = 1;
      PACE_GND_CTRL = 1;
      ATR_PACE_CTRL = 0;
      ATR_GND_CTRL = 1;
      VENT_PACE_CTRL = 0;
      VENT_GND_CTRL = 0;
      Z_ATR_CTRL = 0;
      Z_VENT_CTRL =0;
      FRONTEND_CTRL = 0;
    state Atrial_Pacing
      entry:
      PACING_REF_PWM = atrial_amplitude;
      ATR_CMP_REF_PWM = 70;
      PACE_CHARGE_CTRL = 0;
      PACE_GND_CTRL = 1;
      ATR_PACE_CTRL = 1;
      ATR_GND_CTRL = 0;
      VENT_PACE_CTRL = 0;
      VENT_GND_CTRL = 0;
      Z_ATR_CTRL = 0;
      Z_VENT_CTRL = 0;
    (default) -> AOO.AOO_Charge
    AOO.AOO_Charge -> AOO.Atrial_Pacing : [after(LRI - atrial_pulse_width,msec)]
    AOO.Atrial_Pacing -> AOO.AOO_Charge : [after(atrial_pulse_width,msec)]
  state OFF
    entry:
    ATR_PACE_CTRL = 0;
    VENT_PACE_CTRL = 0;
  state VVIR
    state delay
    state VVI_Charge
      entry:
      PACING_REF_PWM = atrial_amplitude;
      VENT_CMP_REF_PWM = 70;
      PACE_CHARGE_CTRL = 1;
      PACE_GND_CTRL = 1;
      ATR_PACE_CTRL = 0;
      ATR_GND_CTRL = 0;
      VENT_PACE_CTRL = 0;
      VENT_GND_CTRL = 1;
      Z_ATR_CTRL = 0;
      Z_VENT_CTRL =0;
    state sense
      entry:
      FRONTEND_CTRL = 1;
    state inhibited_VRP
    state Ventricular_Pacing
      entry:
      PACING_REF_PWM = atrial_amplitude;
      VENT_CMP_REF_PWM = 70;
      PACE_CHARGE_CTRL = 0;
      PACE_GND_CTRL = 1;
      ATR_PACE_CTRL = 0;
      ATR_GND_CTRL = 0;
      Z_ATR_CTRL = 0;
      Z_VENT_CTRL = 0;
      VENT_PACE_CTRL = 1;
      VENT_GND_CTRL = 0;
    VVIR.delay -> VVIR.sense : [after(VRP - ventricular_pulse_width,msec)]
    (default) -> VVIR.VVI_Charge
    VVIR.sense -> VVIR.delay [order 1] : [VENT_CMP_DETECT == 1]
    VVIR.VVI_Charge -> VVIR.inhibited_VRP
    VVIR.inhibited_VRP -> VVIR.sense : [after(VRP - ventricular_pulse_width,msec)]
    VVIR.sense -> VVIR.Ventricular_Pacing [order 2] : [after(Adaptive_Interval - VRP,msec) && VENT_CMP_DETECT == 0]
    VVIR.Ventricular_Pacing -> VVIR.VVI_Charge : [after(ventricular_pulse_width,msec)]
  state VOOR
    state VOOR_Charge
      entry:
      PACING_REF_PWM = atrial_amplitude;
      VENT_CMP_REF_PWM = 70;
      PACE_CHARGE_CTRL = 1;
      PACE_GND_CTRL = 1;
      ATR_PACE_CTRL = 0;
      ATR_GND_CTRL = 0;
      VENT_PACE_CTRL = 0;
      VENT_GND_CTRL = 1;
      Z_ATR_CTRL = 0;
      Z_VENT_CTRL =0;
      FRONTEND_CTRL = 0;
    state Ventricular_Pacing
      entry:
      PACING_REF_PWM = atrial_amplitude;
      VENT_CMP_REF_PWM = 70;
      PACE_CHARGE_CTRL = 0;
      PACE_GND_CTRL = 1;
      ATR_PACE_CTRL = 0;
      ATR_GND_CTRL = 0;
      Z_ATR_CTRL = 0;
      Z_VENT_CTRL = 0;
      VENT_PACE_CTRL = 1;
      VENT_GND_CTRL = 0;
    (default) -> VOOR_Charge
    VOOR_Charge -> VOOR.Ventricular_Pacing : [after(Adaptive_Interval - ventricular_pulse_width,msec)]
    VOOR.Ventricular_Pacing -> VOOR_Charge : [after(ventricular_pulse_width,msec)]
  state VOO
    state VOO_Charge
      entry:
      PACING_REF_PWM = atrial_amplitude;
      VENT_CMP_REF_PWM = 70;
      PACE_CHARGE_CTRL = 1;
      PACE_GND_CTRL = 1;
      ATR_PACE_CTRL = 0;
      ATR_GND_CTRL = 0;
      VENT_PACE_CTRL = 0;
      VENT_GND_CTRL = 1;
      Z_ATR_CTRL = 0;
      Z_VENT_CTRL =0;
      FRONTEND_CTRL = 0;
    state Ventricular_Pacing
      entry:
      PACING_REF_PWM = atrial_amplitude;
      VENT_CMP_REF_PWM = 70;
      PACE_CHARGE_CTRL = 0;
      PACE_GND_CTRL = 1;
      ATR_PACE_CTRL = 0;
      ATR_GND_CTRL = 0;
      Z_ATR_CTRL = 0;
      Z_VENT_CTRL = 0;
      VENT_PACE_CTRL = 1;
      VENT_GND_CTRL = 0;
    (default) -> VOO_Charge
    VOO_Charge -> VOO.Ventricular_Pacing : [after(LRI - ventricular_pulse_width,msec)]
    VOO.Ventricular_Pacing -> VOO_Charge : [after(ventricular_pulse_width,msec)]
  OFF -> AOOR [order 5] : [mode == 5]
  OFF -> AAIR [order 7] : [mode == 7]
  AAI -> OFF : [mode ~= 3]
  OFF -> AAI [order 1] : [mode == 3]
  AAIR -> OFF : [mode ~= 7]
  AOOR -> OFF : [mode ~= 5]
  (default) -> OFF
  AOO -> OFF : [mode ~= 1]
  OFF -> VVI [order 3] : [mode == 4]
  OFF -> AOO [order 2] : [mode == 1]
  VVI -> OFF : [mode ~= 4]
  VVIR -> OFF : [mode ~= 8]
  VOOR -> OFF : [mode ~= 6]
  OFF -> VOOR [order 6] : [mode == 6]
  VOO -> OFF : [mode ~= 2]
  OFF -> VOO [order 4] : [mode == 2]
  OFF -> VVIR [order 8] : [mode == 8]
  data: PACE_CHARGE_CTRL output; VENT_PACE_CTRL output; ATR_PACE_CTRL output; ATR_GND_CTRL output; VENT_GND_CTRL output; PACE_GND_CTRL output; mode input uint8; LRL input single; LRI input single; URL input single; URI input single; atrial_amplitude input single; ventricular_amplitude input single; Z_VENT_CTRL output; Z_ATR_CTRL output; atrial_pulse_width input single; ventricular_pulse_width input single; ARP input single; VRP input single; PVARP input uint16; VENT_CMP_DETECT input; ATR_CMP_DETECT input; FRONTEND_CTRL output; PACING_REF_PWM output; Adaptive_Interval input single; ATR_CMP_REF_PWM local double; VENT_CMP_REF_PWM local double

== matlab function Assignment1/Parameter Input/VPW Limiter ==
  data: u input; y output
function y = fcn(u)
    if u >= 20
       u = single(20);
    elseif u <= 0
        u = single(0);
    end
y = u;

== matlab function Assignment1/Parameter Input/Atri_Amp Limiter ==
  data: u input; y output
function y = fcn(u)
    if u >= 5
       u = single(5);
    elseif u < 0.5
       u = single(0);
    end
y = u;

== matlab function Assignment1/Parameter Input/LRL Limiter ==
  data: u input; y output
function y = fcn(u)
    if u > 175
       u = single(350);
    elseif u < 30
       u = single(60);
    end
y = 2*u;

== matlab function Assignment1/Parameter Input/ARP Limiter ==
  data: u input; y output
function y = fcn(u)
    if u > 500
       u = single(500);
    elseif u < 150
       u = single(0);
    end
y = u;

== matlab function Assignment1/Parameter Input/VRP Limiter ==
  data: u input; y output
function y = fcn(u)
    if u > 500
       u = single(500);
    elseif u < 150
       u = single(0);
    end
y = u;

== matlab function Assignment1/Parameter Input/URL Limiter ==
  data: u input; y output
function y = fcn(u)
    if u > 175
       u = single(350);
    elseif u < 50
        u = single(100);
    end
y = 2*u;

== matlab function Assignment1/Parameter Input/LRI Function ==
  data: u input; y output single
function y = fcn(u)
y = single(60000/u);

== matlab function Assignment1/Parameter Input/URL Function ==
  data: u input; y output single
function y = fcn(u)
y = single(60000/u);

== stateflow chart Assignment1/Serial Communication ==
  settings: executeAtInitialization=1
  state SET_PARAM
    entry:
    Mode = typecast(rxdata(3), 'uint8');
    lower_rate_limit = typecast(rxdata(4:7), 'single');
    upper_rate_limit = typecast(rxdata(8:11), 'single');
    maximum_sensor_rate = typecast(rxdata(12:15), 'single');
    atrial_amplitude = typecast(rxdata(16:19), 'single');
    ventricular_amplitude = typecast(rxdata(20:23), 'single');
    atrial_pulse_width = typecast(rxdata(24:27), 'single');
    ventricular_pulse_width = typecast(rxdata(28:31), 'single');
    atrial_sensitivity = typecast(rxdata(32:35), 'single');
    ventricular_sensitivity = typecast(rxdata(36:39), 'single');
    ARP = typecast(rxdata(40:43), 'single');
    VRP = typecast(rxdata(44:47), 'single');
    PVARP = typecast(rxdata(48:49), 'uint16');
    activity_threshold = typecast(rxdata(50:53), 'single');
    reaction_time = typecast(rxdata(54:57), 'single');
    response_factor = typecast(rxdata(58:61), 'single');
    recovery_time = typecast(rxdata(62:65), 'single');
  state INITIAL
    entry:
    Mode = 5;
    lower_rate_limit = 30;
    upper_rate_limit = 120;
    maximum_sensor_rate = 120;
    atrial_amplitude = 3.5;
    ventricular_amplitude = 3.5;
    atrial_pulse_width = 20;
    ventricular_pulse_width = 20;
    atrial_sensitivity = 0.75;
    ventricular_sensitivity = 2.5;
    ARP = 250;
    VRP = 320;
    PVARP = 250;
    activity_threshold = 1.6;
    reaction_time = 1;
    response_factor = 80;
    recovery_time = 300;
  state STANDBY
  state ECHO_PARAM
    entry:
    send_params();
  SET_PARAM -> STANDBY
  (default) -> INITIAL
  (junction 13) -> SET_PARAM [order 1] : [rxdata(2)==hex2dec('55')]
  (junction 9) -> STANDBY [order 2]
  INITIAL -> STANDBY
  STANDBY -> (junction 9) : [status == 0]
  (junction 9) -> (junction 13) [order 1] : [rxdata(1)==hex2dec('16')]
  (junction 13) -> ECHO_PARAM [order 2] : [rxdata(2)==hex2dec('22')]
  ECHO_PARAM -> STANDBY
  data: Mode output uint8; lower_rate_limit output single; upper_rate_limit output single; maximum_sensor_rate output single; atrial_amplitude output single; ventricular_amplitude output single; rxdata input uint8; status input uint8 size=1; atrial_pulse_width output single; ventricular_pulse_width output single; atrial_sensitivity output single; ventricular_sensitivity output single; ARP output single; VRP output single; PVARP output uint16; activity_threshold output single; reaction_time output single; response_factor output single; recovery_time output single

== stateflow chart Assignment1/Rate Adaptive Pacing/Adaptive Rate FSM ==
  state wait_increase
  state Init
    adaptive_rate = LRL;
    red_out = 0;
    green_out = 0;
    blue_out = 1;
  state Reached_dessire_rate
    adaptive_rate = desired_rate;
    red_out = 0;
    green_out = 0;
    blue_out = 1;
  state Increase
    adaptive_rate = adaptive_rate + raise_rate/1000;
    red_out = 1;
    green_out = 0;
    blue_out = 0;
  state Decrease
    adaptive_rate = adaptive_rate -  raise_rate/1000;
    red_out = 0;
    green_out = 1;
    blue_out = 0;
  state wait_decrease
  wait_increase -> Increase : [after(reaction_time, msec)]
  Increase -> wait_increase [order 1] : [adaptive_rate < desired_rate]
  (default) -> Init
  Init -> Init [order 2] : [activity_level <= activity_threshold]
  Reached_dessire_rate -> Reached_dessire_rate [order 1] : [activity_level > activity_threshold]
  Init -> Increase [order 1] : [activity_level > activity_threshold]
  Increase -> Reached_dessire_rate [order 2] : [adaptive_rate >= desired_rate]
  Decrease -> Init [order 1] : [adaptive_rate <= LRL && activity_level <= activity_threshold]
  Reached_dessire_rate -> Decrease [order 2] : [activity_level <= activity_threshold]
  Decrease -> Increase [order 3] : [activity_level > activity_threshold]
  Decrease -> wait_decrease [order 2] : [adaptive_rate > LRL && activity_level <= activity_threshold]
  wait_decrease -> Decrease : [after(recovery_time, msec)]
  data: adaptive_rate output single; reaction_time input; recovery_time input; activity_threshold input; LRL input single; raise_rate input single; activity_level input; desired_rate input single; green_out output; red_out output; blue_out output

== matlab function Assignment1/Parameter Input/Vent_Amp Limiter ==
  data: u input; y output
function y = fcn(u)
    if u >= 5
       u = single(5);
    elseif u < 0.5
       u = single(0);
    end
y = u;

== matlab function Assignment1/Parameter Input/Atri_Amp Calculator ==
  data: u input; y output
function y = fcn(u)
y = (u/5)*100;

== matlab function Assignment1/Parameter Input/Vent_Amp Calculator ==
  data: u input; y output
function y = fcn(u)
y = (u/5)*100;

== matlab function Assignment1/Rate Adaptive Pacing/interval converter ==
  data: y output; u input
function y = fcn(u)
y = 60000/single(u);
